simulink model "model4"  (R2022a)
settings: Solver=VariableStepAuto  StartTime=0.0  StopTime=2  MaxStep=0.001  RelTol=1e-3
values from neighbouring files (symbols this model uses):
  A_d = sys_d.A    [config4.m]    (also in config5.m)
  B_d = sys_d.B    [config4.m]    (also in config5.m)
  K_d = K*inv(M)    [config4.m]
  L = (H_z/M_z)'    [task4.m]    (also in task5.m)
  T = 0.2    [config4.m]    (also in config5.m)
  x_0 = [1; 0]    [config4.m]    (also in config5.m)
undefined symbols (not defined in the file or in its folder): A, B, C
settings Model: Creator=Vvlad  LastModifiedBy=Vvlad

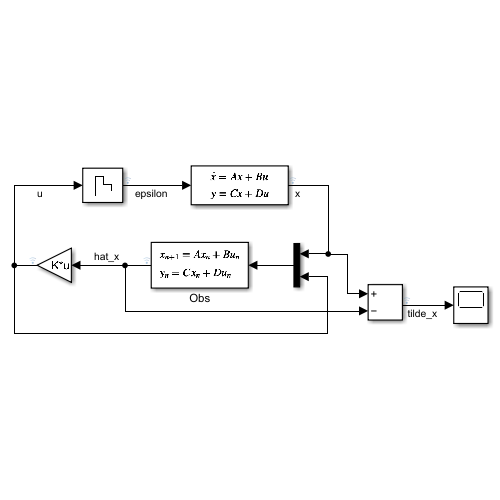
[thumbnail: Simulink's stored preview of the top-level diagram]
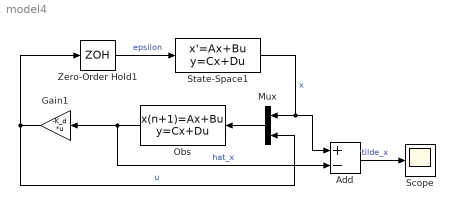
== system model4 ==
  Add : Sum  Inputs=+-
  Gain1 : Gain  Gain=-K_d  Multiplication=Matrix(K*u)
  Mux : Mux  Inputs=2
  Obs : DiscreteStateSpace  A=A_d - L*C  B=[L*C B_d]  C=eye(2)  D=zeros(2, 3)  SampleTime=T
  Scope : Scope
  State-Space1 : StateSpace  A=A  B=B  C=eye(2)  D=[0;0]  InitialCondition=x_0
  Zero-Order Hold1 : ZeroOrderHold  SampleTime=T
  wires:
  Gain1/1 -> Mux/2, Zero-Order Hold1/1  "u"
  Obs/1 -> Add/2, Gain1/1  "hat_x"
  Zero-Order Hold1/1 -> State-Space1/1  "epsilon"
  State-Space1/1 -> Add/1, Mux/1  "x"
  Mux/1 -> Obs/1
  Add/1 -> Scope/1  "tilde_x"
